simulink model "ORC_test_simu_unregSCIG"  (R2018a)
settings: Solver=ode3  StartTime=0.0  StopTime=45  FixedStep=.1  RelTol=1e-4
undefined symbols (not defined in the file or in its folder): A_cond, A_evap, Cx, eff_inverter, eff_pump, eff_pumpdrive, eff_turbine, f_rated, H_wf_init, handle_sink, handle_source, handle_wf, Lr, Ls, m_dot_wf_init, m_dot_wf_max, magCurveV, magCurveX, n_mech_init, n_mech_max, n_mech_min, p_atm, pf_grid, poles, Rr, Rs, Rx, sigbuilder_block, U_cond, U_evap, Vline_rated, Xx
(part 3 of 3)

== matlab function ORC_test_simu_unregSCIG/ORC/Pump/IsentropicPower_pump ==
  data: T_or_H_i input; P_hy output; p_i input; p_o input; m_dot input; T_or_H_o output; T_or_H parameter; isen_eff parameter; fluid parameter
function [ P_hy, T_or_H_o ] = IsentropicPower_block( T_or_H_i, p_i, p_o, m_dot, T_or_H,  isen_eff, fluid)
% function [ P_hy ] = IsentropicPower( T_i, T_o, p_i, p_o, m_dot, fluid, isen_eff )
%EXPANDER Summary of this function
%   This process calculates the mechanical power provided or required by a 
%   generic expander device/system. Turbines and other expanders provide
%   mechanical power while pumps and compressors consume it. This is done
%   by calculating the change in enthalpy of fluid and multipying by the 
%   mass flow rate while entropy remains constant.  Non ideal processes are
%   taken into account through the isentropic efficiency.
% 
% Inputs:
%   T_or_H_i    Input temperature in Kelvin or enthalpy in J/kg
%   p_i         Input pressure of the fluid in Pa
%   p_o         Output temperature of the fluid in Pa
%   m_dot       Mass flow rate of the fluid in kg/s 
%   fluid       Initialzed coolprop fluid handle
%   isen_eff    Isentropic efficiency of the device. Expected range: 0-1
%               This input is optional. If it is not provided then it will 
%               be set to 1, which is the efficiency of an ideal isentropic
%               device where entropy is constant.
%               This value is treated differently depending on if there is
%               an increase or decrease in fluid enthalpy. If the enthalpy
%               decreases (energy is extracted from the system) then the
%               efficiency if multiplied by the change in energy because
%               less energy is extracted than the ideal case. If the
%               enthalpy increases (energy in added to the system) then the
%               efficiency is divided by the change in energy because more
%               energy is required than the ideal case.
%   T_or_H      Logical indicating whether the relavent input and output
%               variables are temperature (1) or enthalpy (0)
% 
% Outputs:
%   P_hy        Hydraulic power exctracted or consumed in W. Positive
%               values indicate the system is providing hydraulic power as
%               a turbine or expander. Negative values indicate the system 
%               is consuming hydraulic power as a compressor or pump.
%   T_or_H_o    Output temperature in Kelvin or enthalpy in J/kg

% This function makes use of the CoolProp wrapper for fluid properties. 
% The high level Matlab wrapper cannot handle vector inputs. There ways to
% make low level calls interfacing with the DLL so many values can be
% determined more quickly, but that is not implented here.
% More information about the Matlab wrapper can be found at
%   http://www.coolprop.org/coolprop/wrappers/MATLAB/index.html
% A list of parameters can be found at 
%   http://www.coolprop.org/coolprop/HighLevelAPI.html#parameter-table
% A list of fluids can be found at 
%   http://www.coolprop.org/fluid_properties/PurePseudoPure.html#list-of-fluids

% initailize certain parameters used to call coolprop library
buffer_size = 255;
ierr = 0;
b = (1:1:buffer_size);
herr= char(b);
coder.extrinsic('calllib') 
coder.extrinsic('libpointer') 

% All the input signals should be the same size, so it shouldn't matter
% which one is used to obtain signal length
var_length = length(T_or_H_i);

% determine input parameter pair indecies for coolprop calls
% [pq_ind,~] = calllib('coolprop','get_input_pair_index','PQ_INPUTS'); %pressure and Mass vapor quality
[pt_ind,~] = calllib('coolprop','get_input_pair_index','PT_INPUTS'); %pressure and temperature
[hp_ind,~] = calllib('coolprop','get_input_pair_index','HmassP_INPUTS'); %Mass specific enthalpy and pressure
[ps_ind,~] = calllib('coolprop','get_input_pair_index','PSmass_INPUTS'); %pressure and Mass specific entropy

% determine output parameter indecies for coolprop calls
[t_ind, ~] = calllib('coolprop','get_param_index','T'); %temperature
[s_ind, ~] = calllib('coolprop','get_param_index','S'); %Mass specific entropy
[h_ind, ~] = calllib('coolprop','get_param_index','Hmass'); %Mass specific enthalpy
% [c_ind, ~] = calllib('coolprop','get_param_index','Cpmass'); %Mass specific constant pressure specific heat

% find pointer location of pressure input and output values
p_i_Ptr = libpointer('doublePtr',p_i);
p_o_Ptr = libpointer('doublePtr',p_o);

% Ensure temperature/enthalpy input variables are delt with appropriately
if T_or_H 
% Assume given temperature values are not at vaporization/condensation.
% Initialize T and H inputs
    T_i = T_or_H_i;
    T_i_Ptr = libpointer('doublePtr',T_i);
    H_i = zeros(var_length,1); % initialized to 0 temporarily
    H_i_Ptr = libpointer('doublePtr',H_i);
% Update values located at Hhi and Hci pointer locations
    calllib('coolprop','AbstractState_update_and_1_out', fluid, pt_ind, p_i_Ptr, T_i_Ptr, var_length, h_ind, H_i_Ptr, ierr,herr,buffer_size);
% Set Hhi & Hci to values stored at pointer location
    H_i = get(H_i_Ptr,'Value');
    
else
% Enthalpy values can be in vaporization/condensation region  
% Initialize H values
    H_i = T_or_H_i;
    H_i_Ptr = libpointer('doublePtr',H_i);

end

% Input entropy in J/kg/K
% Initialize pointer locations for relevant variables
S_i_Ptr = libpointer('doublePtr', zeros(var_length,1)); 
% Update values at S_i pointer location
calllib('coolprop','AbstractState_update_and_1_out', fluid, hp_ind, H_i_Ptr, p_i_Ptr, var_length, s_ind, S_i_Ptr, ierr,herr,buffer_size);
% Set S_i to values stored at pointer location
% S_i = get(S_i_Ptr,'Value');

% Ideal Output entropy is equal to input entropy 
% Ideal Output enthalpy in J/kg and temperature
H_o_ideal = zeros(var_length,1);
H_o_ideal_Ptr = libpointer('doublePtr',H_o_ideal);
% Update values located at Hhi and Hci pointer locations
calllib('coolprop','AbstractState_update_and_1_out', fluid, ps_ind, p_o_Ptr, S_i_Ptr, var_length, h_ind, H_o_ideal_Ptr, ierr,herr,buffer_size);
% Set H_o_ideal to values stored at pointer location
H_o_ideal = get(H_o_ideal_Ptr,'Value');

% Calculate Ideal power consumed/provided
P_ideal = m_dot.*(H_i - H_o_ideal);

% Initialize hydrolic power variable
P_hy = zeros(var_length,1);
%   If positive then the system is providing power as a turbine
%   or expander.
%   This means the actual power provided is less than the ideal power
P_hy(P_ideal > 0) = isen_eff.*P_ideal(P_ideal > 0);

%   If negative then the system is consuming power as a
%   compressor or pump.
%   This means the actual power consumed is greater than the ideal power.
P_hy(P_ideal < 0) = P_ideal(P_ideal < 0)./isen_eff;

% Set output enthalpy
H_o = H_i - P_hy./m_dot;
H_o_Ptr = libpointer('doublePtr',H_o);

% Ensure temperature/enthalpy input variables are delt with appropriately
if T_or_H 
% Assume given temperature values are not at vaporization/condensation
    T_or_H_o = zeros(var_length,1);
    T_or_H_o_Ptr = libpointer('doublePtr',T_or_H_o);
    calllib('coolprop','AbstractState_update_and_1_out', fluid, hp_ind, H_o_Ptr, p_o_Ptr, var_length, t_ind, T_or_H_o_Ptr, ierr,herr,buffer_size);
    T_or_H_o = get(T_or_H_o_Ptr,'Value');
    
else
% Enthalpy values can be in vaporization/condensation region    
    T_or_H_o = H_o;
end
end

== matlab function ORC_test_simu_unregSCIG/ORC/hp2t ==
  data: temperature output; enthalpy input; pressure input; fluid_handle parameter
function temperature  = hp2t(enthalpy,pressure, fluid_handle)
%HP2T Summary of this function goes here
%   This function takes caluculates the temperature of a fluid based off of
%   its enthalpy and pressure using the Cool Prob library. The fluid handle
%   must already be generated and input in order to calculate the output
%   values.

buffer_size = 255;
ierr = 0;
b = (1:1:buffer_size);
herr= char(b);
coder.extrinsic('calllib') 
coder.extrinsic('libpointer') 

[hp_ind,~] = calllib('coolprop','get_input_pair_index','HmassP_INPUTS'); %Mass specific enthalpy and pressure
[t_ind, ~] = calllib('coolprop','get_param_index','T'); %temperature

var_len = length(pressure);
pressurePtr = libpointer('doublePtr',pressure);
enthaplyPtr = libpointer('doublePtr',enthalpy);
temperature = zeros(var_len,1);
temperaturePtr = libpointer('doublePtr',temperature);

calllib('coolprop','AbstractState_update_and_1_out', fluid_handle, hp_ind, enthaplyPtr, pressurePtr, var_len, t_ind, temperaturePtr, ierr,herr,buffer_size);

temperature = get(temperaturePtr,'Value');

end

== matlab function ORC_test_simu_unregSCIG/ORC/hp2t1 ==
  data: temperature output; enthalpy input; pressure input; fluid_handle parameter
function temperature  = hp2t(enthalpy,pressure, fluid_handle)
%HP2T Summary of this function goes here
%   This function takes caluculates the temperature of a fluid based off of
%   its enthalpy and pressure using the Cool Prob library. The fluid handle
%   must already be generated and input in order to calculate the output
%   values.

buffer_size = 255;
ierr = 0;
b = (1:1:buffer_size);
herr= char(b);
coder.extrinsic('calllib') 
coder.extrinsic('libpointer') 

[hp_ind,~] = calllib('coolprop','get_input_pair_index','HmassP_INPUTS'); %Mass specific enthalpy and pressure
[t_ind, ~] = calllib('coolprop','get_param_index','T'); %temperature

var_len = length(pressure);
pressurePtr = libpointer('doublePtr',pressure);
enthaplyPtr = libpointer('doublePtr',enthalpy);
temperature = zeros(var_len,1);
temperaturePtr = libpointer('doublePtr',temperature);

calllib('coolprop','AbstractState_update_and_1_out', fluid_handle, hp_ind, enthaplyPtr, pressurePtr, var_len, t_ind, temperaturePtr, ierr,herr,buffer_size);

temperature = get(temperaturePtr,'Value');

end

== matlab function ORC_test_simu_unregSCIG/ORC/hp2t2 ==
  data: temperature output; enthalpy input; pressure input; fluid_handle parameter
function temperature  = hp2t(enthalpy,pressure, fluid_handle)
%HP2T Summary of this function goes here
%   This function takes caluculates the temperature of a fluid based off of
%   its enthalpy and pressure using the Cool Prob library. The fluid handle
%   must already be generated and input in order to calculate the output
%   values.

buffer_size = 255;
ierr = 0;
b = (1:1:buffer_size);
herr= char(b);
coder.extrinsic('calllib') 
coder.extrinsic('libpointer') 

[hp_ind,~] = calllib('coolprop','get_input_pair_index','HmassP_INPUTS'); %Mass specific enthalpy and pressure
[t_ind, ~] = calllib('coolprop','get_param_index','T'); %temperature

var_len = length(pressure);
pressurePtr = libpointer('doublePtr',pressure);
enthaplyPtr = libpointer('doublePtr',enthalpy);
temperature = zeros(var_len,1);
temperaturePtr = libpointer('doublePtr',temperature);

calllib('coolprop','AbstractState_update_and_1_out', fluid_handle, hp_ind, enthaplyPtr, pressurePtr, var_len, t_ind, temperaturePtr, ierr,herr,buffer_size);

temperature = get(temperaturePtr,'Value');

end

== matlab function ORC_test_simu_unregSCIG/ORC/hp2t3 ==
  data: temperature output; enthalpy input; pressure input; fluid_handle parameter
function temperature  = hp2t(enthalpy,pressure, fluid_handle)
%HP2T Summary of this function goes here
%   This function takes caluculates the temperature of a fluid based off of
%   its enthalpy and pressure using the Cool Prob library. The fluid handle
%   must already be generated and input in order to calculate the output
%   values.

buffer_size = 255;
ierr = 0;
b = (1:1:buffer_size);
herr= char(b);
coder.extrinsic('calllib') 
coder.extrinsic('libpointer') 

[hp_ind,~] = calllib('coolprop','get_input_pair_index','HmassP_INPUTS'); %Mass specific enthalpy and pressure
[t_ind, ~] = calllib('coolprop','get_param_index','T'); %temperature

var_len = length(pressure);
pressurePtr = libpointer('doublePtr',pressure);
enthaplyPtr = libpointer('doublePtr',enthalpy);
temperature = zeros(var_len,1);
temperaturePtr = libpointer('doublePtr',temperature);

calllib('coolprop','AbstractState_update_and_1_out', fluid_handle, hp_ind, enthaplyPtr, pressurePtr, var_len, t_ind, temperaturePtr, ierr,herr,buffer_size);

temperature = get(temperaturePtr,'Value');

end

== matlab function ORC_test_simu_unregSCIG/ORC/hp2t4 ==
  data: temperature output; enthalpy input; pressure input; fluid_handle parameter
function temperature  = hp2t(enthalpy,pressure, fluid_handle)
%HP2T Summary of this function goes here
%   This function takes caluculates the temperature of a fluid based off of
%   its enthalpy and pressure using the Cool Prob library. The fluid handle
%   must already be generated and input in order to calculate the output
%   values.

buffer_size = 255;
ierr = 0;
b = (1:1:buffer_size);
herr= char(b);
coder.extrinsic('calllib') 
coder.extrinsic('libpointer') 

[hp_ind,~] = calllib('coolprop','get_input_pair_index','HmassP_INPUTS'); %Mass specific enthalpy and pressure
[t_ind, ~] = calllib('coolprop','get_param_index','T'); %temperature

var_len = length(pressure);
pressurePtr = libpointer('doublePtr',pressure);
enthaplyPtr = libpointer('doublePtr',enthalpy);
temperature = zeros(var_len,1);
temperaturePtr = libpointer('doublePtr',temperature);

calllib('coolprop','AbstractState_update_and_1_out', fluid_handle, hp_ind, enthaplyPtr, pressurePtr, var_len, t_ind, temperaturePtr, ierr,herr,buffer_size);

temperature = get(temperaturePtr,'Value');

end

== matlab function ORC_test_simu_unregSCIG/ORC/hp2t5 ==
  data: temperature output; enthalpy input; pressure input; fluid_handle parameter
function temperature  = hp2t(enthalpy,pressure, fluid_handle)
%HP2T Summary of this function goes here
%   This function takes caluculates the temperature of a fluid based off of
%   its enthalpy and pressure using the Cool Prob library. The fluid handle
%   must already be generated and input in order to calculate the output
%   values.

buffer_size = 255;
ierr = 0;
b = (1:1:buffer_size);
herr= char(b);
coder.extrinsic('calllib') 
coder.extrinsic('libpointer') 

[hp_ind,~] = calllib('coolprop','get_input_pair_index','HmassP_INPUTS'); %Mass specific enthalpy and pressure
[t_ind, ~] = calllib('coolprop','get_param_index','T'); %temperature

var_len = length(pressure);
pressurePtr = libpointer('doublePtr',pressure);
enthaplyPtr = libpointer('doublePtr',enthalpy);
temperature = zeros(var_len,1);
temperaturePtr = libpointer('doublePtr',temperature);

calllib('coolprop','AbstractState_update_and_1_out', fluid_handle, hp_ind, enthaplyPtr, pressurePtr, var_len, t_ind, temperaturePtr, ierr,herr,buffer_size);

temperature = get(temperaturePtr,'Value');

end

== matlab function ORC_test_simu_unregSCIG/ORC/pt2h ==
  data: fluid_handle parameter; pressure input; enthalpy output; temperature input
function enthalpy  = pt2h(fluid_handle,pressure,temperature)
%PT2H Summary of this function goes here
%   This function takes caluculates the enthalpy of a fluid based off of
%   its temperature and pressure using the Cool Prob library. The fluid 
%   handle must already be generated and input in order to calculate the 
%   output values.

buffer_size = 255;
ierr = 0;
b = (1:1:buffer_size);
herr= char(b);
coder.extrinsic('calllib') 
coder.extrinsic('libpointer') 

[pt_ind,~] = calllib('coolprop','get_input_pair_index','PT_INPUTS'); %Mass specific enthalpy and pressure
[h_ind, ~] = calllib('coolprop','get_param_index','Hmass'); %temperature

var_len = length(pressure);
pressurePtr = libpointer('doublePtr',pressure);
temperaturePtr  = libpointer('doublePtr',temperature);
enthalpy = zeros(var_len,1);
enthaplyPtr = libpointer('doublePtr',enthalpy);

calllib('coolprop','AbstractState_update_and_1_out', fluid_handle, pt_ind, pressurePtr, temperaturePtr, var_len, h_ind, enthaplyPtr, ierr,herr,buffer_size);

enthalpy = get(enthaplyPtr,'Value');

end

== matlab function ORC_test_simu_unregSCIG/ORC/pt2h2 ==
  data: fluid_handle parameter; pressure input; enthalpy output; temperature input
function enthalpy  = pt2h(fluid_handle,pressure,temperature)
%PT2H Summary of this function goes here
%   This function takes caluculates the enthalpy of a fluid based off of
%   its temperature and pressure using the Cool Prob library. The fluid 
%   handle must already be generated and input in order to calculate the 
%   output values.

buffer_size = 255;
ierr = 0;
b = (1:1:buffer_size);
herr= char(b);
coder.extrinsic('calllib') 
coder.extrinsic('libpointer') 

[pt_ind,~] = calllib('coolprop','get_input_pair_index','PT_INPUTS'); %Mass specific enthalpy and pressure
[h_ind, ~] = calllib('coolprop','get_param_index','Hmass'); %temperature

var_len = length(pressure);
pressurePtr = libpointer('doublePtr',pressure);
temperaturePtr  = libpointer('doublePtr',temperature);
enthalpy = zeros(var_len,1);
enthaplyPtr = libpointer('doublePtr',enthalpy);

calllib('coolprop','AbstractState_update_and_1_out', fluid_handle, pt_ind, pressurePtr, temperaturePtr, var_len, h_ind, enthaplyPtr, ierr,herr,buffer_size);

enthalpy = get(enthaplyPtr,'Value');

end

== matlab function ORC_test_simu_unregSCIG/Inverter ==
  data: eff input; Pin input; Pout output; Ploss output
function [ Pout, Ploss ] = Inverter_Simple(eff, Pin)
% function [ Pdc, Ploss ] = Voltage_Source_Inverter_Simple(Pload, Qload, Vdc, Vac, eff, method_flag )
                            
%INVERTER Summary of this function goes here
%   This function simulates a very simple three phase voltage source 
%   inverter for an energy balance microgrid model. For a given load, input
%   and output voltage levels, and efficiency, the scripts will calculated
%   the power comsumptions seen by the DC source as well as the power loss
%   in the inverter.

% Active Power out = Active Power in * efficiency
Pout = Pin.*eff;

% loss is the difference in power
Ploss = Pin - Pout;

end

== matlab function ORC_test_simu_unregSCIG/Generator/MATLAB Function ==
  data: n_mech input; P_load_out output; P_loss output; Q_loss output; P_load_in input; Vline input; P_mech_needed output; f_e output; Xm output; Vline_out output; f_rated parameter; poles parameter; K_b parameter; K_w parameter; R1 parameter; L1 parameter; R2 parameter; L2 parameter; Cx parameter; magCurveX parameter; magCurveV parameter
function [ P_load_out, P_loss, Q_loss, P_mech_needed, f_e, Xm, Vline_out] = SCIG_Ouazenne_it( n_mech, P_load_in, Vline, f_rated, poles, K_b, K_w, R1, L1, R2, L2, Cx, magCurveX, magCurveV)
%SCIG_ENERGY_BALANCE Summary of this function goes here 
%   This function calcluates the active power (P_loss) losses of a 3-phase 
%   squirrel cage induction generator (SCIG). Also calclulated is the
%   reactive power loss (Q_loss). Induction machines always consume Q
%   (negative Q_out) and the excitation capacitance generates Q (positive
%   Q_out).

%   Circuit diagram of an Asynchronous machine. 
%      Iin>   Ix         I1>        Im        I2>
%              v      R1     jw*X1   v     R2     jw*X2
%     0--------|-----RRRR----XXXX----|----RRRR----XXXX----|
%              |                    E|                    |
%     +        R  Rx               |-|-|                  |
%              R                   |   |                  R
%     Vph      |               Rm  R   X   jw*Xm          R  R2(1-slip)/slip
%              |                   R   X                  R
%     -       CCC  1/jw*Cx         |   |                  R
%              |                   |-|-|                  |
%              |                     |                    |  
%     0--------|---------------------|--------------------|
  
% Inputs:
%   P_load      Three phase active load power in W
%   Q_load      Three phase reactive load power in VAR
%   n_mech      Angular velocity of rotor in rpm
%   f_rated     Rated synchronous frequency in Hz
%   Vline_rated Rated line voltage in V
%   poles       Number of poles
%   K_b         Bearing coefficient 
%   K_w         Windage coefficient
%   R1          Stator resistance in ohm
%   L1          Stator inductance in H
%   R2          Rotor resistance in ohm
%   L2          Rotor inductance in H
%   Rm          Magnetizing resistance of the core in ohm
%   Lm          Magnetizing inductance of the core in L
%   Cx          External Excitation capacitance in F
%
% Outputs:
%   P_loss
%   Q_loss
%   Vph
%   P_mech      Mech power to rotor (P_mech = w_mech*Torque)

var_length = size(n_mech);
P_load_out = zeros(var_length);
% Q_out = zeros(var_length);
P_loss = zeros(var_length);
Q_loss = zeros(var_length);
f_e = zeros(var_length);
Xm = zeros(var_length);
Vline_out = zeros(var_length);


n_synchRated = f_rated*120/poles;
b = n_mech./n_synchRated;

% The mechanical angular velocity
w_mech = 2*pi*n_mech/60;

% calculate reactive impedance from inductance values (X = w*L) and 
% capacitance value (X = 1/(w*C)) at rated frequencies
X1 = 2*pi*f_rated.*L1;
X2 = 2*pi*f_rated.*L2;
Xx = 1./(Cx*2*pi*f_rated);

% calculate friction and windage losses
P_bearing = K_b .* w_mech;
P_windage = K_w .* w_mech.^2;

% calculated the impedance of the load based off power consumed at rated
% line to line voltage
Z_load = LoadImpedance(P_load_in, 0, Vline);
R_load = real(Z_load);

% Calcluate coefficients used to calculated the operating frequency
% relative to the rated frequency. These coefficients can be found in the
% appendix of Analysis of the Isolated Inducution Generator by Ouazenne and
% McPherson.  Note in the text Q2 and Q3 both have a typo which has been
% corrected here.
if R_load < inf
    Rtemp = R1 + R_load;
    
    Q0 = -b*R2*(Rtemp/R_load)^2;
    Q1 = R2*(Rtemp/R_load)^2 + Rtemp*(R2/R_load)^2 + b^2*Rtemp*(X2/R_load)^2;
    Q2 = -2*b*Rtemp*(X2/R_load)^2 - b*R2*((R1/Xx)^2 + (X1/R_load)^2 - 2*(X1/Xx));
    Q3 = R2*((X1/R_load)^2 + (R1/Xx)^2 - 2*(X1/Xx)) + Rtemp*(X2/R_load)^2 + R1*(R2/Xx)^2 + b^2*R1*(X2/Xx)^2;
    Q5 = R2*(X1/Xx)^2 + R1*(X2/Xx)^2;
    Q4 = -b*(Q5 + R1*(X2/Xx)^2);

else
    Q0 = -b*R2;
    Q1 = R2;
    Q2 = - b*R2*((R1/Xx)^2 - 2*(X1/Xx));
    Q3 = R2*((R1/Xx)^2 - 2*(X1/Xx)) + R1*(R2/Xx)^2 + b^2*R1*(X2/Xx);
    Q5 = R2*(X1/Xx)^2 + R1*(X2/Xx)^2;
    Q4 = -b*(Q5 + R1*(X2/Xx)^2);
end

% Calculate all the roots based from the coeffecients
aroots = roots([Q5 Q4 Q3 Q2 Q1 Q0]);

% Ouazzene and McPherson state there should only be one real root
a = real(aroots(end));
% a = aroots(~imag(aroots))
% a = .95;

% Calculate the series equivalent of load and ext. excitation capacitance
RL = R_load*Xx^2/(a*(a^2*R_load^2 + Xx^2));
XL = R_load^2*Xx/(a^2*R_load^2 + Xx^2);

% % calculate the operating frquency
f_e = a*f_rated;

% Calculate impedance of the core base of Ouazenne and McPherson
if R_load < inf
    Xm = ((RL + R1/a)*(X2^2 + (R2/(a-b))^2))/((R2/(a-b))*(X1-XL) - X2*(RL + R1/a));
else
    Xm = ((R1/a)*(X2^2 + (R2/(a-b))^2))/((R2/(a-b))*(X1 - Xx/a^2) - R1*X2/a);
end

% from Xm and magnatization curve calculate internal voltage magnitude
E_f = interp1(magCurveX,magCurveV,Xm,'linear');
% E_f = 240;

% calcluate phase voltage magnitude
if R_load < inf
    Vph = a*E_f/sqrt((1-a^2*(X1/Xx))^2 + a^2*((X1/R_load)^2 + (R1/Xx)^2) + (1 + R1/R_load)^2 - 1);
else
    Vph = a*E_f/sqrt((1-a^2*(X1/Xx))^2 + (a*R1/Xx)^2);
end

Vline_out = Vph*sqrt(3);

% calculate slip from electrical frequency and rotor speed relative to
% rated values
slip = (a-b)/a;


% recalculate reactive impedances for operating frequency
X1 = 2*pi*f_e.*L1;
X2 = 2*pi*f_e.*L2;
Xx = 1./(Cx*2*pi*f_e);
Xm = Xm*f_e/f_rated;

% calculate stator, rotor, core, and excitation per-unit impedances
Z_stator = R1 + 1i*X1;   % R1 and X1 in series
% Z_core = 1./(1./Rm + 1./(1i*Xm));   % Rm and Xm in parallel
Z_core = 1i*Xm;
Z_rotor = R2./slip + 1i*X2;   % R2/slip and X2 in series
Z_machine = Z_stator + 1./(1./Z_core + 1./Z_rotor);
Z_excite = Xx/(1i);   

% Calculate stator current 
I1 = Vph/Z_machine;

% Calculate excitation current
Ix = Vph./Z_excite;

% Calculate internal voltage
E = Vph - I1*Z_stator;

% Calculate magnetizing current
Im = E./Z_core;

% Calculate rotor current
I2 = E./Z_rotor;

% Calculate load current
Iload = Vph./Z_load;

 
% Calculate active and reactive power losses in the asynch machine
Q_loss_rotor = 3*abs(I2).^2.*X2;
P_RCL = 3*abs(I2).^2.*R2;

Q_loss_stator = 3*abs(I1).^2.*X1;
P_SCL = 3*abs(I1).^2.*R1;

Q_loss_core = 3*abs(E).^2./(Xm);
P_core =0;% 3*abs(E).^2./Rm;

if any(Ix)
%     Sometimes when there is an infinite impedance matlab will calculate
%     NaN even though there is 0 current. This if/else ensures the power
%     calculations result in 0 when current is 0.
    Q_loss_excitation = -3*abs(Ix).^2.*(Xx);
else
    Q_loss_excitation = 0;
end

 
% Calculate total real and reactive powers. Reactive power is only
% consumed not generated therefore Q_out should be negative.
Q_loss(:) = (Q_loss_core + Q_loss_rotor + Q_loss_stator);% + Q_loss.excitation;
% P_out = P_conv -(P_excitation + P_RCL + P_SCL + P_core);

% Output real losses in stucture
P_loss_mech = P_bearing + P_windage;
P_loss_copper = P_RCL + P_SCL;
P_loss_core = P_core;
P_loss(:) = P_bearing + P_windage + P_RCL + P_SCL + P_core;

P_load_out(:) = real(3*abs(Vph)^2/conj(Z_load));
P_conv = -3.*abs(I2).^2.*R2.*(1-slip)./slip;
P_mech_needed = P_conv + P_bearing + P_windage;
% Q_out(:) = zeros(var_length);%Q_loss + Q_loss_excitation;
end
%
